simulink model "Hit"  (R2013b)
settings: Solver=ode15s  StartTime=0.0  StopTime=1  MaxStep=0.8  RelTol=1e-3
undefined symbols (not defined in the file): sigbuilder_block
libraries: fl_lib x15, nesl_utility x6
Description:
  | Mechanical System with Translational Hard Stop
  | 
  | This example shows two masses interacting through a hard stop. The left mass
  | is driven by an ideal velocity source in such a way that plotting
  | the displacement of the second mass against the displacement of the first mass
  | produces a typical hysteresis curve.
  | 
  | 
  | Copyright 2008-2013 The MathWorks, Inc.
settings Model: ExtModeAutoUpdateStatusClock=off  Creator=MathWorks  LastModifiedBy=Eugenio
settings DataIOCC: SignalLoggingSaveFormat=ModelDataLogs
settings OptimizationCC: ExpressionDepthLimit=2147483647  InitFltsAndDblsToZero=on
settings DebuggingCC: SaveWithParameterizedLinksMsg=none  SignalResolutionControl=TryResolveAllWithWarning  MultiTaskDSMMsg=warning  FcnCallInpInsideContextMsg=UseLocalSettings  StateNameClashWarn=warning
settings GRTTargetCC: TargetFcnLib=ansi_tfl_tmw.mat  CombineOutputUpdateFcns=off  GRTInterface=on

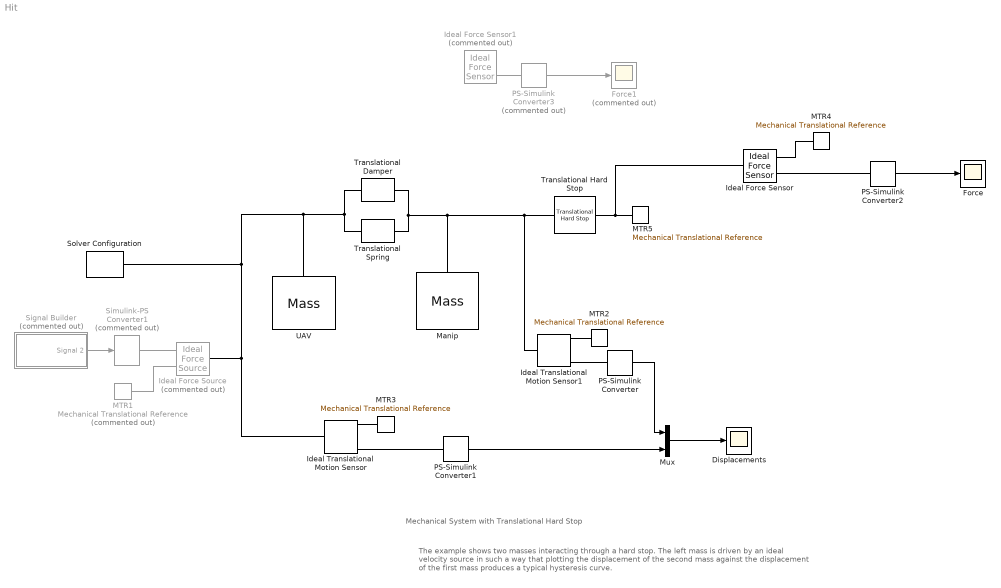
== system Hit ==
  note: The example shows two masses interacting through a hard stop. The left mass is driven by an ideal velocity source in such a way
      | that plotting the displacement of the second mass against the displacement of the first mass produces a typical hysteresis curve.
  note: Mechanical System with Translational Hard Stop
  Displacements : Scope
      settings: TimeRange=40  YMin=-2  YMax=1.5  MaxDataPoints=50000
  Force : Scope
      settings: TimeRange=40  YMin=-2  YMax=1.5  MaxDataPoints=50000
  Force1 : Scope  Commented=on
      settings: TimeRange=40  YMin=-2  YMax=1.5  SaveName=ScopeData2  MaxDataPoints=50000
  Ideal Force Sensor : fl_lib/Mechanical/Mechanical Sensors/Ideal Force Sensor  v_Log=off  f_Log=off  LocalVarNames=|v|f  LocalVarDescs=|v|f  LocalVarLogging=[0 0]
  Ideal Force Sensor1 : fl_lib/Mechanical/Mechanical Sensors/Ideal Force Sensor  Commented=on  v_Log=off  f_Log=off  LocalVarNames=|v|f  LocalVarDescs=|v|f  LocalVarLogging=[0 0]
  Ideal Force Source : fl_lib/Mechanical/Mechanical Sources/Ideal Force Source  Commented=on  v_Log=off  f_Log=off  LocalVarNames=|v|f  LocalVarDescs=|v|f  LocalVarLogging=[0 0]
  Ideal Translational Motion Sensor : fl_lib/Mechanical/Mechanical Sensors/Ideal Translational Motion Sensor  Tag=Factory Generic  offset=-0.6 m  v_Log=off  f_Log=off  x_Log=off  LocalVarNames=|v|f|x  LocalVarDescs=|v|f|x  LocalVarLogging=[]
  Ideal Translational Motion Sensor1 : fl_lib/Mechanical/Mechanical Sensors/Ideal Translational Motion Sensor  Tag=Factory Generic  offset=0 m  v_Log=off  f_Log=off  x_Log=off  LocalVarNames=|v|f|x  LocalVarDescs=|v|f|x  LocalVarLogging=[]
  MTR1 : fl_lib/Mechanical/Translational Elements/Mechanical Translational Reference  Tag=Factory Generic  Commented=on  f_Log=off  LocalVarNames=|f  LocalVarDescs=|f  LocalVarLogging=[]
  MTR{2..5} (4 alike) : fl_lib/Mechanical/Translational Elements/Mechanical Translational Reference  Tag=Factory Generic  f_Log=off  LocalVarNames=|f  LocalVarDescs=|f  LocalVarLogging=[]
  Manip : fl_lib/Mechanical/Translational Elements/Mass  Tag=Factory Generic  mass=0.1 kg  initial_velocity=10 m/s  f_Log=off  LocalVarNames=|force|velocity  LocalVarDescs=|Inertia force (N)|Mass absolute velocity (m/s)  LocalVarLogging=[0 0]
  Mux : Mux  Inputs=2
  PS-Simulink Converter : nesl_utility/PS-Simulink Converter  PhysicalDomain=network_engine_domain  SubClassName=ps_output  LeftPortType=input  RightPortType=output  PseudoPeriodic=off  Frequencies=[]  Unit=1  AffineConversion=off
  PS-Simulink Converter1 : nesl_utility/PS-Simulink Converter  PhysicalDomain=network_engine_domain  SubClassName=ps_output  LeftPortType=input  RightPortType=output  PseudoPeriodic=off  Frequencies=[]  Unit=1  AffineConversion=off
  PS-Simulink Converter2 : nesl_utility/PS-Simulink Converter  PhysicalDomain=network_engine_domain  SubClassName=ps_output  LeftPortType=input  RightPortType=output  PseudoPeriodic=off  Frequencies=[]  Unit=1  AffineConversion=off
  PS-Simulink Converter3 : nesl_utility/PS-Simulink Converter  Commented=on  PhysicalDomain=network_engine_domain  SubClassName=ps_output  LeftPortType=input  RightPortType=output  PseudoPeriodic=off  Frequencies=[]  Unit=1  AffineConversion=off
  Signal Builder : Subsystem  Tag=STV Subsys  Commented=on  LoadFcn=sigbuilder_block('load');  StartFcn=sigbuilder_block('start');  StopFcn=sigbuilder_block('stop');  ClipboardFcn=sigbuilder_block('clipboard');  mask(Sigbuilder block){}
      mask help: Simulink:masks:SigbuilderBlock_MD
      mask init:
      | if ~strcmp(get_param(bdroot(gcbh),'SimulationStatus'),'stopped') tuvar = sigbuilder_block('maskInit'); end
      settings: CopyFcn=sigbuilder_block('copy');  DeleteFcn=sigbuilder_block('delete');  ModelCloseFcn=sigbuilder_block('modelClose');  PreSaveFcn=sigbuilder_block('preSave');  PauseFcn=sigbuilder_block('pause');  ContinueFcn=sigbuilder_block('continue');  NameChangeFcn=sigbuilder_block('namechange');  OpenFcn=sigbuilder_block('open',[55.5 114 549 400.5 ]);  CloseFcn=sigbuilder_block('close');
      mask Display: plot(0, 0, 100, 100,[2, 2, 32, 32, 2], [68, 8, 8, 68, 68],[32, 2], [38, 38], [32, 19, 2],[53, 60, 44], [32, 17, 17, 2],[16, 16, 31, 31]);txt = getActiveGroup(gcbh);text(2, 100, txt,'verticalAlignment', 'top');
  Simulink-PS Converter1 : nesl_utility/Simulink-PS Converter  Commented=on  PhysicalDomain=network_engine_domain  SubClassName=ps_input  LeftPortType=input  RightPortType=output  PseudoPeriodic=off  Frequencies=[]  NoiseDistribution=none  NoiseParameters=[]  Unit=1  AffineConversion=off  InputFiltering=off  SimscapeFilterOrder=1  InputFilterTimeConstant=0.001  UdotUserProvided=1
  Solver Configuration : nesl_utility/Solver Configuration  PhysicalDomain=network_engine_domain  SubClassName=solver  LeftPortType=input  RightPortType=generic  Accelerate=off  Tones=[]  Harmonics=[]  SimulateNoise=off  Profile=off  UseLocalSampling=off  EnableSwitchedLinearOptims=on  FrequencyDomain=off  UseCCode=off  RelTol=0.001  AbsTol=1e-06  MinStep=1e-09  ToWorkspace=off  DoDC=off  ResidualTolerance=1e-9  UseLocalSolver=off  LocalSolverChoice=NE_BACKWARD_EULER_ADVANCER  LocalSolverSampleTime=.001  DoFixedCost=off  MaxNonlinIter=3  MaxModeIter=2  LinearAlgebra=Sparse  DelaysMemoryBudget=1024
  Translational Hard Stop : fl_lib/Mechanical/Translational Elements/Translational Hard Stop  Tag=Factory Generic  upper_bnd=1 m  lower_bnd=-100 m  stiff_up=1e+06 N/m  stiff_low=1e+04 N/m  D_up=0.1 N/(m/s)  D_low=0.8 N/(m/s)  initial_position=0 m  f_Log=off  v_Log=off  x_Log=off  LocalVarNames=|contact_force|rel_displacement  LocalVarDescs=|Contact force (N)|Slider-case relative displacement (m)  LocalVarLogging=[0 0]
  Translational Damper : fl_lib/Mechanical/Translational Elements/Translational Damper  D=10 N/(m/s)  f_Log=off  v_Log=off  LocalVarNames=|f|v  LocalVarDescs=|f|v  LocalVarLogging=[0 0]
  Translational Spring : fl_lib/Mechanical/Translational Elements/Translational Spring  spr_rate=200 N/m  init_def=0 m  f_Log=off  v_Log=off  x_Log=off  LocalVarNames=|f|v|x  LocalVarDescs=|f|v|x  LocalVarLogging=[0 0 0]
  UAV : fl_lib/Mechanical/Translational Elements/Mass  Tag=Factory Generic  mass=1 kg  initial_velocity=10 m/s  f_Log=off  LocalVarNames=|force|velocity  LocalVarDescs=|Inertia force (N)|Mass absolute velocity (m/s)  LocalVarLogging=[0 0]
  wires:
  PS-Simulink Converter/1 -> Mux/1
  PS-Simulink Converter1/1 -> Mux/2
  Mux/1 -> Displacements/1
  Signal Builder/1(Signal 2) -> Simulink-PS Converter1/1
  PS-Simulink Converter2/1 -> Force/1
  PS-Simulink Converter3/1 -> Force1/1
  connections:
  MTR5/LConn1 -- Ideal Force Sensor/LConn1 -- Translational Hard Stop/RConn1
  Ideal Translational Motion Sensor1/RConn3 -- PS-Simulink Converter/LConn1
  Ideal Translational Motion Sensor/RConn3 -- PS-Simulink Converter1/LConn1
  MTR2/LConn1 -- Ideal Translational Motion Sensor1/RConn1
  MTR3/LConn1 -- Ideal Translational Motion Sensor/RConn1
  Translational Damper/LConn1 -- Translational Hard Stop/LConn1 -- Ideal Translational Motion Sensor1/LConn1 -- Manip/LConn1 -- Translational Spring/LConn1
  Translational Damper/RConn1 -- Solver Configuration/RConn1 -- Ideal Force Source/LConn1 -- Ideal Translational Motion Sensor/LConn1 -- UAV/LConn1 -- Translational Spring/RConn1
  MTR1/LConn1 -- Ideal Force Source/RConn2
  Simulink-PS Converter1/RConn1 -- Ideal Force Source/RConn1
  Ideal Force Sensor/RConn2 -- PS-Simulink Converter2/LConn1
  Ideal Force Sensor/RConn1 -- MTR4/LConn1
  PS-Simulink Converter3/LConn1 -- Ideal Force Sensor1/RConn2

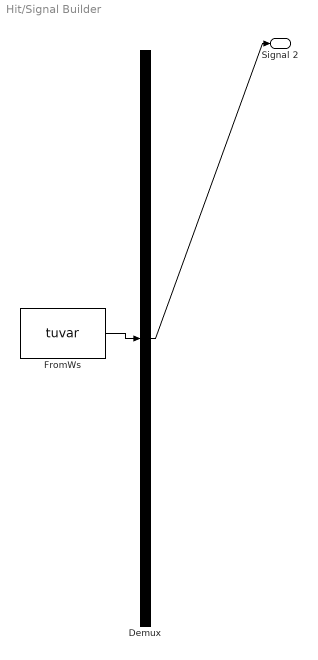
== system Hit/Signal Builder ==
  Demux : Demux  Tag=STV Demux  Outputs=1
  FromWs : FromWorkspace  Tag=STV FromWs  VariableName=tuvar  SampleTime=0
      SigBuilderData=|
      | common.afterFinalStr = 'Extrapolate'
      | common.sampleTime = 0
      | dataSet.timeRange = [0 10]
      | dataSet.name = 'Group 1'
      | sbobj.Groups.Name = 'Group 1'
      | sbobj.Groups.Signals.Name = 'Signal 2'
      | sbobj.Groups.Signals.XData = [0 1.2 1.2 1.8 1.8 3 3 4.52 4.52 10]
      | sbobj.Groups.Signals.YData = [9.95 8.62 7.36 4.64 -0.6 -0.66 3.22 3.22 -0.02 0.04]
  Signal 2 : Outport  Tag=STV Outport
  wires:
  FromWs/1 -> Demux/1
  Demux/1 -> Signal 2/1
